simulink model "encoder_decoder_fcn"  (R2021a)
settings: Solver=VariableStepAuto  StartTime=0.0  StopTime=0.1*8  RelTol=1e-3
libraries: simulink x2, simulink_extras x1
settings Model: Creator=kjartan  LastModifiedBy=kjartan

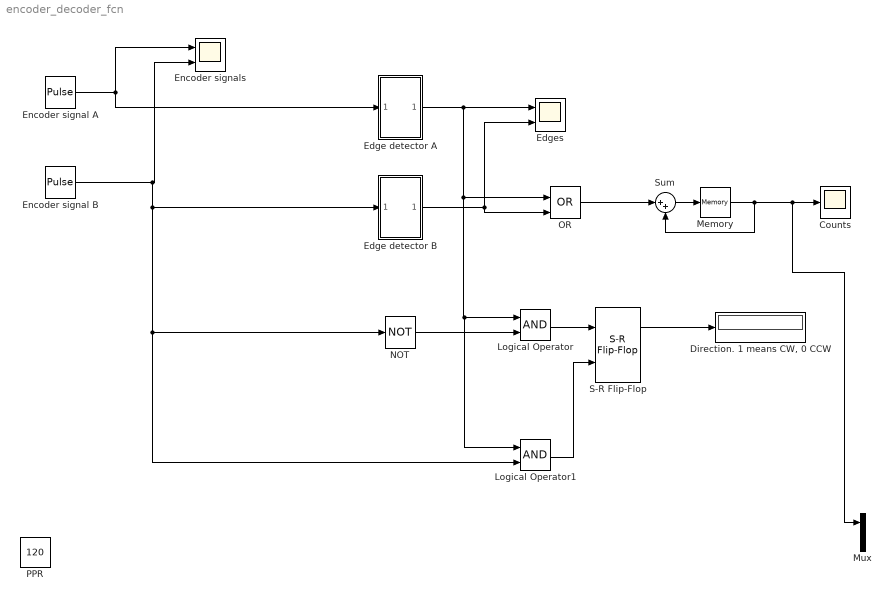
== system encoder_decoder_fcn ==
  Counts : Scope
  "Direction. 1 means CW, 0 CCW" : Display
  Edge detector A : Subsystem
  Edge detector B : Subsystem
  Edges : Scope  NumInputPorts=2
  "Encoder signal A " : DiscretePulseGenerator  PulseType=Time based  Period=0.1  PulseWidth=50
  Encoder signal B : DiscretePulseGenerator  PulseType=Time based  Period=0.1  PulseWidth=50  PhaseDelay=0.1/4
  Encoder signals : Scope  NumInputPorts=2
  Logical Operator : Logic  AllPortsSameDT=off  OutDataTypeStr=boolean
  Logical Operator1 : Logic  AllPortsSameDT=off  OutDataTypeStr=boolean
  Memory : Memory
  Mux : Mux  Inputs=2
  NOT : Logic  Operator=NOT  IconShape=distinctive  AllPortsSameDT=off  OutDataTypeStr=boolean
  OR : Logic  Operator=OR  IconShape=distinctive  AllPortsSameDT=off  OutDataTypeStr=fixdt(1,16)
  PPR : Constant  Value=120
  S-R Flip-Flop : simulink_extras/Flip Flops/S-R Flip-Flop  initial_condition=0
  Sum : Sum  Inputs=|++
  wires:
  "Encoder signal A "/1 -> Encoder signals/1, Edge detector A/1(In1)
  Encoder signal B/1 -> Logical Operator1/2, NOT/1, Edge detector B/1(In1), Encoder signals/2
  Edge detector B/1(Out1) -> OR/2, Edges/2
  NOT/1 -> Logical Operator/2
  Logical Operator/1 -> S-R Flip-Flop/1
  Logical Operator1/1 -> S-R Flip-Flop/2
  S-R Flip-Flop/1 -> "Direction. 1 means CW, 0 CCW"/1
  Edge detector A/1(Out1) -> Logical Operator1/1, Logical Operator/1, OR/1, Edges/1
  Memory/1 -> Sum/2, Mux/1, Counts/1
  OR/1 -> Sum/1
  Sum/1 -> Memory/1

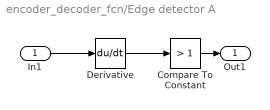
== system encoder_decoder_fcn/Edge detector A ==
  In1 : Inport
  Compare To Constant : simulink/Logic and Bit Operations/Compare To Constant  relop=>  const=1  OutDataTypeStr=boolean
  Derivative : Derivative  CoefficientInTFapproximation=1e6
  Out1 : Outport
  wires:
  Derivative/1 -> Compare To Constant/1
  In1/1 -> Derivative/1
  Compare To Constant/1 -> Out1/1

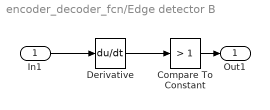
== system encoder_decoder_fcn/Edge detector B ==
  In1 : Inport
  Compare To Constant : simulink/Logic and Bit Operations/Compare To Constant  relop=>  const=1  OutDataTypeStr=boolean
  Derivative : Derivative  CoefficientInTFapproximation=1e6
  Out1 : Outport
  wires:
  Compare To Constant/1 -> Out1/1
  In1/1 -> Derivative/1
  Derivative/1 -> Compare To Constant/1
